simulink model "TriTiltPro_V3"  (R2019a)
settings: Solver=ode15s  StartTime=0.0  StopTime=1  RelTol=1e-3  EnableMultiTasking=on
undefined symbols (not defined in the file or in its folder): magnitude, sigbuilder_block, X, Y, Z
libraries: sm_lib x405, nesl_utility x28, simulink x13, fl_lib x7, fl_ps_legacy_lib x6, sharedtransform x1, Multibody_Multiphysics_Lib x1
(part 9 of 9)

== system TriTiltPro_V3/ASingle-Tilt Tricopter 3D Model/Tricopter/Frame/FrameA/plain_washer_10669_type_nl_iso_15_solid1_1_RIGID ==
  ReferenceFrame : sm_lib/Frames and Transforms/Reference Frame
  Solid : sm_lib/Body Elements/Solid  InertiaType=Custom  Mass=4.3196898986859697e-05  MassUnits=kg  CenterOfMass=[0.3937007874015751 0.27559055118110243 2.6256152004553557]  CenterOfMassUnits=in  MomentsOfInertia=[3.1106329160175101e-07 3.1106329160175101e-07 6.1096736198012081e-07]  MomentsOfInertiaUnits=kg*in^2  ProductsOfInertia=[0 0 0]  ProductsOfInertiaUnits=kg*in^2  BasedOnType=Density  Density=1000  DensityUnits=kg/(m^3)  DoExposeReferenceFrame=on  SerializedFrames=<Frames/>  GraphicType=FromGeometry  MarkerShape=Sphere  MarkerSize=10  MarkerSizeUnits=m  GraphicVisPropType=SimpleVisualProperties  GraphicDiffuseColor=[0.792156862745098 0.81960784313725488 0.93333333333333335]  GraphicSpecularColor=[0.5 0.5 0.5 1.0]  GraphicAmbientColor=[0.15 0.15 0.15 1.0]  GraphicEmissiveColor=[0.0 0.0 0.0 1.0]  GraphicShininess=75  GraphicOpacity=1  GeometryShape=FromFile  RectangleSize=[1 1]  RectangleSizeUnits=m  BrickDimensions=[1 1 1]  BrickDimensionUnits=m  CylinderRadius=1  CylinderRadiusUnits=m  CylinderLength=1  CylinderLengthUnits=m  SphereRadius=1  SphereRadiusUnits=m  EllipsoidRadii=[1 1 1]  EllipsoidRadiiUnits=m  ExtrusionCrossSection=[1 1; -1 1; -1 -1; 1 -1]  ExtrusionCrossSectionUnits=m  ExtrusionLength=1  ExtrusionLengthUnits=m  PolygonNumSides=3  PolygonOuterRadius=1  PolygonOuterRadiusUnits=m  ExtGeomFileType=STL  ExtGeomFileName=plain washer 10669 type nl_iso-15-solid1_Default_sldprt.STL  ExtGeomFileUnits=in  RevolutionCrossSection=[1 1; 1 -1; 2 -1; 2 1]  RevolutionCrossSectionUnits=m  RevolutionExtent=Full  RevolutionAngle=180  RevolutionAngleUnits=deg
  F : PMIOPort  Side=Left
  connections:
  Solid/RConn1 -- ReferenceFrame/RConn1 -- F/RConn1

== system TriTiltPro_V3/ASingle-Tilt Tricopter 3D Model/Tricopter/Frame/FrameA/plain_washer_10669_type_nl_iso_16_solid1_1_RIGID ==
  ReferenceFrame : sm_lib/Frames and Transforms/Reference Frame
  Solid : sm_lib/Body Elements/Solid  InertiaType=Custom  Mass=4.3196898986859697e-05  MassUnits=kg  CenterOfMass=[0.39370078740157505 0.27559055118110237 2.1138041768333089]  CenterOfMassUnits=in  MomentsOfInertia=[3.1106329160175085e-07 3.1106329160175095e-07 6.109673619801206e-07]  MomentsOfInertiaUnits=kg*in^2  ProductsOfInertia=[0 0 0]  ProductsOfInertiaUnits=kg*in^2  BasedOnType=Density  Density=1000  DensityUnits=kg/(m^3)  DoExposeReferenceFrame=on  SerializedFrames=<Frames/>  GraphicType=FromGeometry  MarkerShape=Sphere  MarkerSize=10  MarkerSizeUnits=m  GraphicVisPropType=SimpleVisualProperties  GraphicDiffuseColor=[0.792156862745098 0.81960784313725488 0.93333333333333335]  GraphicSpecularColor=[0.5 0.5 0.5 1.0]  GraphicAmbientColor=[0.15 0.15 0.15 1.0]  GraphicEmissiveColor=[0.0 0.0 0.0 1.0]  GraphicShininess=75  GraphicOpacity=1  GeometryShape=FromFile  RectangleSize=[1 1]  RectangleSizeUnits=m  BrickDimensions=[1 1 1]  BrickDimensionUnits=m  CylinderRadius=1  CylinderRadiusUnits=m  CylinderLength=1  CylinderLengthUnits=m  SphereRadius=1  SphereRadiusUnits=m  EllipsoidRadii=[1 1 1]  EllipsoidRadiiUnits=m  ExtrusionCrossSection=[1 1; -1 1; -1 -1; 1 -1]  ExtrusionCrossSectionUnits=m  ExtrusionLength=1  ExtrusionLengthUnits=m  PolygonNumSides=3  PolygonOuterRadius=1  PolygonOuterRadiusUnits=m  ExtGeomFileType=STL  ExtGeomFileName=plain washer 10669 type nl_iso-16-solid1_Default_sldprt.STL  ExtGeomFileUnits=in  RevolutionCrossSection=[1 1; 1 -1; 2 -1; 2 1]  RevolutionCrossSectionUnits=m  RevolutionExtent=Full  RevolutionAngle=180  RevolutionAngleUnits=deg
  F : PMIOPort  Side=Left
  connections:
  Solid/RConn1 -- ReferenceFrame/RConn1 -- F/RConn1

== system TriTiltPro_V3/ASingle-Tilt Tricopter 3D Model/Tricopter/Frame/FrameA/socket_head_cap_screw_iso_7_solid1_1_RIGID ==
  ReferenceFrame : sm_lib/Frames and Transforms/Reference Frame
  Solid : sm_lib/Body Elements/Solid  InertiaType=Custom  Mass=0.00020359080750969805  MassUnits=kg  CenterOfMass=[-0.39370078740157455 0.27559055118110221 2.3901587604267629]  CenterOfMassUnits=in  MomentsOfInertia=[1.6336628993777264e-05 1.6336628993777264e-05 6.509380073908462e-07]  MomentsOfInertiaUnits=kg*in^2  ProductsOfInertia=[0 0 0]  ProductsOfInertiaUnits=kg*in^2  BasedOnType=Density  Density=1000  DensityUnits=kg/(m^3)  DoExposeReferenceFrame=on  SerializedFrames=<Frames/>  GraphicType=FromGeometry  MarkerShape=Sphere  MarkerSize=10  MarkerSizeUnits=m  GraphicVisPropType=SimpleVisualProperties  GraphicDiffuseColor=[0.792156862745098 0.81960784313725488 0.93333333333333335]  GraphicSpecularColor=[0.5 0.5 0.5 1.0]  GraphicAmbientColor=[0.15 0.15 0.15 1.0]  GraphicEmissiveColor=[0.0 0.0 0.0 1.0]  GraphicShininess=75  GraphicOpacity=1  GeometryShape=FromFile  RectangleSize=[1 1]  RectangleSizeUnits=m  BrickDimensions=[1 1 1]  BrickDimensionUnits=m  CylinderRadius=1  CylinderRadiusUnits=m  CylinderLength=1  CylinderLengthUnits=m  SphereRadius=1  SphereRadiusUnits=m  EllipsoidRadii=[1 1 1]  EllipsoidRadiiUnits=m  ExtrusionCrossSection=[1 1; -1 1; -1 -1; 1 -1]  ExtrusionCrossSectionUnits=m  ExtrusionLength=1  ExtrusionLengthUnits=m  PolygonNumSides=3  PolygonOuterRadius=1  PolygonOuterRadiusUnits=m  ExtGeomFileType=STL  ExtGeomFileName=socket head cap screw_iso-7-solid1_Default_sldprt.STL  ExtGeomFileUnits=in  RevolutionCrossSection=[1 1; 1 -1; 2 -1; 2 1]  RevolutionCrossSectionUnits=m  RevolutionExtent=Full  RevolutionAngle=180  RevolutionAngleUnits=deg
  F : PMIOPort  Side=Left
  connections:
  Solid/RConn1 -- ReferenceFrame/RConn1 -- F/RConn1

== system TriTiltPro_V3/ASingle-Tilt Tricopter 3D Model/Tricopter/Left Rotor/ESC2/T-W Linear Characteristic ==
  Tdemand : Inport
  Gain : Gain  Gain=1000
  MaxSpeed(rpm) : Constant  Value=1000
  Sum : Sum  Inputs=|+-
  Wdemand : Outport
  wires:
  Sum/1 -> Wdemand/1
  Gain/1 -> Sum/2
  MaxSpeed(rpm)/1 -> Sum/1
  Tdemand/1 -> Gain/1

== system TriTiltPro_V3/ASingle-Tilt Tricopter 3D Model/Tricopter/Left Rotor/ESC2/Torque-Speed DC Servomotor Linear Model ==
  Tmax : Inport
  Wmax : Inport  Port=2
  Wmotor : Inport  Port=3
  SpeedControl : Subsystem
  TorqueControl : Subsystem
  Tmotor : PMIOPort  Side=Right
  wires:
  SpeedControl/1(WmotorIn) -> TorqueControl/3(Wmotor)
  Wmotor/1 -> SpeedControl/1(Wmotor)
  Tmax/1 -> SpeedControl/2(Tmax), TorqueControl/1(Tmax)
  Wmax/1 -> SpeedControl/3(Wmax), TorqueControl/2(Wmax)
  connections:
  SpeedControl/LConn1 -- Tmotor/RConn1 -- TorqueControl/RConn1

== system TriTiltPro_V3/ASingle-Tilt Tricopter 3D Model/Tricopter/Left Rotor/ESC2/Torque-Speed DC Servomotor Linear Model/SpeedControl ==
  Wmotor : Inport
  Tmax : Inport  Port=2
  Wmax : Inport  Port=3
  PID Controller : simulink/Continuous/PID Controller  Controller=PID  Form=Parallel  TimeDomain=Continuous-time  SampleTime=-1  IntegratorMethod=Forward Euler  FilterMethod=Forward Euler  ControllerParametersSource=internal  P=0.00844997126405228  I=0.0134253378530917  D=-0.000204446558053762  UseFilter=on  N=30.4158154473445  TunerSelectOption=Transfer Function Based (PID Tuner App)  InitialConditionSource=internal  InitialConditionForIntegrator=0  InitialConditionForFilter=0  DifferentiatorICPrevScaledInput=0  ExternalReset=none  TrackingMode=off  Kt=1  LimitOutput=off  UpperSaturationLimit=inf  LowerSaturationLimit=-inf  LinearizeAsGain=on  AntiWindupMode=none  Kb=1  POutMin=[]  POutMax=[]  IOutMin=[]  IOutMax=[]  DOutMin=[]  DOutMax=[]  NOutMin=[]  NOutMax=[]  SumOutMin=[]  SumOutMax=[]  SaturationOutMin=[]  SaturationOutMax=[]  PParamMin=[]  PParamMax=[]  IParamMin=[]  IParamMax=[]  DParamMin=[]  DParamMax=[]  NParamMin=[]  NParamMax=[]  KbParamMin=[]  KbParamMax=[]  KtParamMin=[]  KtParamMax=[]  KbOutMin=[]  KbOutMax=[]  KtOutMin=[]  KtOutMax=[]  IntegratorOutMin=[]  IntegratorOutMax=[]  FilterOutMin=[]  FilterOutMax=[]  SumI1OutMin=[]  SumI1OutMax=[]  SumI2OutMin=[]  SumI2OutMax=[]  SumI3OutMin=[]  SumI3OutMax=[]  SumI4OutMin=[]  SumI4OutMax=[]  SumDOutMin=[]  SumDOutMax=[]  DifferentiatorOutMin=[]  DifferentiatorOutMax=[]  FilterDiffOutCoefMin=[]  FilterDiffOutCoefMax=[]  ReciprocalOutMin=[]  ReciprocalOutMax=[]  SumDenOutMin=[]  SumDenOutMax=[]  SumNumOutMin=[]  SumNumOutMax=[]  DivideOutMin=[]  DivideOutMax=[]  IntegratorContinuousStateAttributes=''  IntegratorStateMustResolveToSignalObject=off  IntegratorRTWStateStorageClass=Auto  FilterContinuousStateAttributes=''  FilterStateMustResolveToSignalObject=off  FilterRTWStateStorageClass=Auto  ParallelPVariant=InternalParameters  IdealPVariant=Disabled  IVariant=InternalParameters  DVariant=InternalParameters  IntegratorVariant=Continuous  SatVariant=Disabled  AWVariant=Passthrough  PCopyVariant=Disabled  TRVariant=Disabled  FdbkBlocksVariant=Forward  IdealPFdbkVariant=Disabled  SatFdbkVariant=Disabled  DerivativeFilterVariant=ContFilter  NVariant=InternalParameters  NCopyVariant=Disabled  FilterICVariant=InternalICsFilter  IntegratorICVariant=InternalICs  ExternalResetVariant=Disabled  TRSumVariant=Passthrough  SumFdbkVariant=Disabled  SumVariant=Sum_PID
  PS Product1 : fl_ps_legacy_lib/Legacy Physical Signals/Functions/PS Product
      settings: SourceProductName=Simscape  SourceProductBaseCode=SS
  PS-Simulink Converter1 : nesl_utility/PS-Simulink Converter  PhysicalDomain=network_engine_domain  SubClassName=ps_output  LeftPortType=input  RightPortType=output  PseudoPeriodic=off  Frequencies=[]  Unit=rpm  AffineConversion=off
  SpeedContol : Subsystem
  SpeedConv : nesl_utility/Simulink-PS Converter  PhysicalDomain=network_engine_domain  SubClassName=ps_input  LeftPortType=input  RightPortType=output  PseudoPeriodic=off  Frequencies=[]  NoiseDistribution=none  NoiseParameters=[]  Unit=rpm  AffineConversion=off  FilteringAndDerivatives=zero  SimscapeFilterOrder=1  InputFilterTimeConstant=0.001  UdotUserProvided=1
  Sum1 : Sum  Inputs=|+-
  Tmotor : PMIOPort  Side=Left
  WmotorIn : Outport
  wires:
  Wmax/1 -> Sum1/1
  Tmax/1 -> SpeedContol/1(Tmax)
  Wmotor/1 -> Sum1/2
  Sum1/1 -> PID Controller/1
  PID Controller/1 -> SpeedConv/1
  PS-Simulink Converter1/1 -> WmotorIn/1
  connections:
  SpeedContol/RConn1 -- Tmotor/RConn1
  PS-Simulink Converter1/LConn1 -- PS Product1/RConn1
  PS Product1/LConn2 -- SpeedContol/RConn2
  SpeedConv/RConn1 -- PS Product1/LConn1

== system TriTiltPro_V3/ASingle-Tilt Tricopter 3D Model/Tricopter/Left Rotor/ESC2/Torque-Speed DC Servomotor Linear Model/TorqueControl ==
  Tmax : Inport
  Wmax : Inport  Port=2
  Wmotor : Inport  Port=3
  PID Controller1 : simulink/Continuous/PID Controller  Commented=on  Controller=PID  Form=Parallel  TimeDomain=Continuous-time  SampleTime=-1  IntegratorMethod=Forward Euler  FilterMethod=Forward Euler  ControllerParametersSource=internal  P=0.719361444578474  I=3441.18525946798  D=0.0000001  UseFilter=on  N=100  TunerSelectOption=Transfer Function Based (PID Tuner App)  InitialConditionSource=internal  InitialConditionForIntegrator=0  InitialConditionForFilter=0  DifferentiatorICPrevScaledInput=0  ExternalReset=none  TrackingMode=off  Kt=1  LimitOutput=on  UpperSaturationLimit=1  LowerSaturationLimit=0  LinearizeAsGain=on  AntiWindupMode=clamping  Kb=1  POutMin=[]  POutMax=[]  IOutMin=[]  IOutMax=[]  DOutMin=[]  DOutMax=[]  NOutMin=[]  NOutMax=[]  SumOutMin=[]  SumOutMax=[]  SaturationOutMin=[]  SaturationOutMax=[]  PParamMin=[]  PParamMax=[]  IParamMin=[]  IParamMax=[]  DParamMin=[]  DParamMax=[]  NParamMin=[]  NParamMax=[]  KbParamMin=[]  KbParamMax=[]  KtParamMin=[]  KtParamMax=[]  KbOutMin=[]  KbOutMax=[]  KtOutMin=[]  KtOutMax=[]  IntegratorOutMin=[]  IntegratorOutMax=[]  FilterOutMin=[]  FilterOutMax=[]  SumI1OutMin=[]  SumI1OutMax=[]  SumI2OutMin=[]  SumI2OutMax=[]  SumI3OutMin=[]  SumI3OutMax=[]  SumI4OutMin=[]  SumI4OutMax=[]  SumDOutMin=[]  SumDOutMax=[]  DifferentiatorOutMin=[]  DifferentiatorOutMax=[]  FilterDiffOutCoefMin=[]  FilterDiffOutCoefMax=[]  ReciprocalOutMin=[]  ReciprocalOutMax=[]  SumDenOutMin=[]  SumDenOutMax=[]  SumNumOutMin=[]  SumNumOutMax=[]  DivideOutMin=[]  DivideOutMax=[]  IntegratorContinuousStateAttributes=''  IntegratorStateMustResolveToSignalObject=off  IntegratorRTWStateStorageClass=Auto  FilterContinuousStateAttributes=''  FilterStateMustResolveToSignalObject=off  FilterRTWStateStorageClass=Auto  ParallelPVariant=InternalParameters  IdealPVariant=Disabled  IVariant=InternalParameters  DVariant=InternalParameters  IntegratorVariant=Continuous  SatVariant=Enabled  AWVariant=ContClampingParallel  PCopyVariant=Disabled  TRVariant=Disabled  FdbkBlocksVariant=Forward  IdealPFdbkVariant=Disabled  SatFdbkVariant=Disabled  DerivativeFilterVariant=ContFilter  NVariant=InternalParameters  NCopyVariant=Disabled  FilterICVariant=InternalICsFilter  IntegratorICVariant=InternalICs  ExternalResetVariant=Disabled  TRSumVariant=Passthrough  SumFdbkVariant=Disabled  SumVariant=Sum_PID
  PS Product : fl_ps_legacy_lib/Legacy Physical Signals/Functions/PS Product
      settings: SourceProductName=Simscape  SourceProductBaseCode=SS
  TorqueControl : Subsystem
  TorqueMaxConv : nesl_utility/Simulink-PS Converter  PhysicalDomain=network_engine_domain  SubClassName=ps_input  LeftPortType=input  RightPortType=output  PseudoPeriodic=off  Frequencies=[]  NoiseDistribution=none  NoiseParameters=[]  Unit=N*m  AffineConversion=off  FilteringAndDerivatives=zero  SimscapeFilterOrder=1  InputFilterTimeConstant=0.001  UdotUserProvided=1
  Tmotor : PMIOPort  Side=Right
  wires:
  Wmotor/1 -> TorqueControl/2(Wmotor)
  Tmax/1 -> TorqueMaxConv/1
  Wmax/1 -> TorqueControl/1(Wmax)
  connections:
  PS Product/RConn1 -- Tmotor/RConn1
  TorqueControl/RConn1 -- PS Product/LConn2
  PS Product/LConn1 -- TorqueMaxConv/RConn1

== system TriTiltPro_V3/ASingle-Tilt Tricopter 3D Model/Tricopter/Left Rotor/ESC2/Torque-Speed DC Servomotor Linear Model/SpeedControl/SpeedContol ==
  Tmax : Inport
  1 : fl_lib/Physical Signals/Sources/PS Constant  constant=1
  PS Divide1 : fl_ps_legacy_lib/Legacy Physical Signals/Functions/PS Divide
      settings: SourceProductName=Simscape  SourceProductBaseCode=SS
  PS Subtract : fl_ps_legacy_lib/Legacy Physical Signals/Functions/PS Subtract
      settings: SourceProductName=Simscape  SourceProductBaseCode=SS
  TorqueMaxConv2 : nesl_utility/Simulink-PS Converter  PhysicalDomain=network_engine_domain  SubClassName=ps_input  LeftPortType=input  RightPortType=output  PseudoPeriodic=off  Frequencies=[]  NoiseDistribution=none  NoiseParameters=[]  Unit=N*m  AffineConversion=off  FilteringAndDerivatives=zero  SimscapeFilterOrder=1  InputFilterTimeConstant=0.001  UdotUserProvided=1
  Tmotor : PMIOPort  Side=Right
  1-Tratio : PMIOPort  Port=2  Side=Right
  wires:
  Tmax/1 -> TorqueMaxConv2/1
  connections:
  TorqueMaxConv2/RConn1 -- PS Divide1/LConn2
  PS Divide1/LConn1 -- Tmotor/RConn1
  1/RConn1 -- PS Subtract/LConn1
  PS Subtract/LConn2 -- PS Divide1/RConn1
  1-Tratio/RConn1 -- PS Subtract/RConn1

== system TriTiltPro_V3/ASingle-Tilt Tricopter 3D Model/Tricopter/Left Rotor/ESC2/Torque-Speed DC Servomotor Linear Model/TorqueControl/TorqueControl ==
  Wmax : Inport
  Wmotor : Inport  Port=2
  1 : fl_lib/Physical Signals/Sources/PS Constant  constant=1
  PS Divide1 : fl_ps_legacy_lib/Legacy Physical Signals/Functions/PS Divide
      settings: SourceProductName=Simscape  SourceProductBaseCode=SS
  PS Subtract : fl_ps_legacy_lib/Legacy Physical Signals/Functions/PS Subtract
      settings: SourceProductName=Simscape  SourceProductBaseCode=SS
  SpeedConv : nesl_utility/Simulink-PS Converter  PhysicalDomain=network_engine_domain  SubClassName=ps_input  LeftPortType=input  RightPortType=output  PseudoPeriodic=off  Frequencies=[]  NoiseDistribution=none  NoiseParameters=[]  Unit=rpm  AffineConversion=off  FilteringAndDerivatives=zero  SimscapeFilterOrder=1  InputFilterTimeConstant=0.001  UdotUserProvided=1
  SpeedConv1 : nesl_utility/Simulink-PS Converter  PhysicalDomain=network_engine_domain  SubClassName=ps_input  LeftPortType=input  RightPortType=output  PseudoPeriodic=off  Frequencies=[]  NoiseDistribution=none  NoiseParameters=[]  Unit=rpm  AffineConversion=off  FilteringAndDerivatives=zero  SimscapeFilterOrder=1  InputFilterTimeConstant=0.001  UdotUserProvided=1
  1-Wratio : PMIOPort  Side=Right
  wires:
  Wmotor/1 -> SpeedConv1/1
  Wmax/1 -> SpeedConv/1
  connections:
  SpeedConv1/RConn1 -- PS Divide1/LConn1
  PS Divide1/LConn2 -- SpeedConv/RConn1
  1/RConn1 -- PS Subtract/LConn1
  1-Wratio/RConn1 -- PS Subtract/RConn1
  PS Subtract/LConn2 -- PS Divide1/RConn1

== matlab function TriTiltPro_V3/ASingle-Tilt Tricopter 3D Model/MATLAB Function ==
  data: u1 input; y output; u2 input; u3 input
function y = fcn(u1,u2,u3)
%#codegen

y = sqrt(u1.^2 + u2.^2 + u3.^2);

== matlab function TriTiltPro_V3/ASingle-Tilt Tricopter 3D Model/6DOF + World/Ground Contact and Maximum Saturation/MATLAB Function ==
  data: z input; force output; v input
function force = fcn(z,v)
%#codegen

%% parameters
upbound = 2.5;
lobound = 0.0;
upstiff = 10e-6;
lostiff = 2e6;
updamp = 1.5e4;
lodamp = 150;

%% equations
if (z > upbound)
    force = -1 * (upstiff * (z - upbound) + updamp * v);
elseif (z < lobound)
    force = abs(lostiff * (z - lobound) + lodamp * v);
else
    force = 0;
end
